simulink model "SF049A_LoaMgr"  (R2013b)
settings: Solver=FixedStepDiscrete  SolverMode=SingleTasking  StartTime=0.0  StopTime=1  FixedStep=0.002  RelTol=1e-3
values from neighbouring files (symbols this model uses):
  CURRMEASLOAMTGTNMASK_CNT_U08 = DataDict.Constant    [SF049A_LoaMgr_DataDict.m]
  IVTRLOAMTGTNMASK_CNT_U08 = DataDict.Constant    [SF049A_LoaMgr_DataDict.m]
  LOAMAXSLEW_ULSPERSEC_F32 = DataDict.Constant    [SF049A_LoaMgr_DataDict.m]
  LoaMgrCurrIvtrMtgtnRate = DataDict.Calibration    [SF049A_LoaMgr_DataDict.m]
  LoaMgrCurrIvtrMtgtnSca = DataDict.Calibration    [SF049A_LoaMgr_DataDict.m]
  LoaMgrCurrIvtrMtgtnScaZeroEna = DataDict.Calibration    [SF049A_LoaMgr_DataDict.m]
  LoaMgrCurrMeasIdptSig0Resp = DataDict.Calibration    [SF049A_LoaMgr_DataDict.m]
  LoaMgrCurrMeasIdptSig1Resp = DataDict.Calibration    [SF049A_LoaMgr_DataDict.m]
  LoaMgrCurrMeasIdptSig2Resp = DataDict.Calibration    [SF049A_LoaMgr_DataDict.m]
  LoaMgrCurrMeasIdptSigFltThd = DataDict.Calibration    [SF049A_LoaMgr_DataDict.m]
  LoaMgrCurrMeasMtgtnRate = DataDict.Calibration    [SF049A_LoaMgr_DataDict.m]
  LoaMgrCurrMeasMtgtnSca = DataDict.Calibration    [SF049A_LoaMgr_DataDict.m]
  LoaMgrCurrMeasMtgtnScaZeroEna = DataDict.Calibration    [SF049A_LoaMgr_DataDict.m]
  LoaMgrFadeOutStRate = DataDict.Calibration    [SF049A_LoaMgr_DataDict.m]
  LoaMgrHwTqIdptSig0NoTqLoaResp = DataDict.Calibration    [SF049A_LoaMgr_DataDict.m]
  LoaMgrHwTqIdptSig1NoTqLoaResp = DataDict.Calibration    [SF049A_LoaMgr_DataDict.m]
  LoaMgrHwTqIdptSig2Resp = DataDict.Calibration    [SF049A_LoaMgr_DataDict.m]
  LoaMgrHwTqIdptSig4Resp = DataDict.Calibration    [SF049A_LoaMgr_DataDict.m]
  LoaMgrHwTqIdptSigFltThd = DataDict.Calibration    [SF049A_LoaMgr_DataDict.m]
  LoaMgrHwTqLoaAvlResp = DataDict.Calibration    [SF049A_LoaMgr_DataDict.m]
  LoaMgrIvtrIdptSig0Resp = DataDict.Calibration    [SF049A_LoaMgr_DataDict.m]
  LoaMgrIvtrIdptSig1Resp = DataDict.Calibration    [SF049A_LoaMgr_DataDict.m]
  LoaMgrIvtrIdptSig2Resp = DataDict.Calibration    [SF049A_LoaMgr_DataDict.m]
  LoaMgrIvtrIdptSigFltThd = DataDict.Calibration    [SF049A_LoaMgr_DataDict.m]
  LoaMgrIvtrMtgtnRate = DataDict.Calibration    [SF049A_LoaMgr_DataDict.m]
  LoaMgrIvtrMtgtnSca = DataDict.Calibration    [SF049A_LoaMgr_DataDict.m]
  LoaMgrIvtrMtgtnScaZeroEna = DataDict.Calibration    [SF049A_LoaMgr_DataDict.m]
  LoaMgrLimdStRate = DataDict.Calibration    [SF049A_LoaMgr_DataDict.m]
  LoaMgrLimdStSca = DataDict.Calibration    [SF049A_LoaMgr_DataDict.m]
  LoaMgrMotAgAvlSnsrlsResp = DataDict.Calibration    [SF049A_LoaMgr_DataDict.m]
  LoaMgrMotAgIdptSig0NoSnsrlsResp = DataDict.Calibration    [SF049A_LoaMgr_DataDict.m]
  LoaMgrMotAgIdptSig1NoSnsrlsResp = DataDict.Calibration    [SF049A_LoaMgr_DataDict.m]
  LoaMgrMotAgIdptSig2Resp = DataDict.Calibration    [SF049A_LoaMgr_DataDict.m]
  LoaMgrMotAgIdptSig3Resp = DataDict.Calibration    [SF049A_LoaMgr_DataDict.m]
  LoaMgrMotAgIdptSigFltThd = DataDict.Calibration    [SF049A_LoaMgr_DataDict.m]
  LoaMgrMotAgMtgtnRate = DataDict.Calibration    [SF049A_LoaMgr_DataDict.m]
  LoaMgrMotAgMtgtnSca = DataDict.Calibration    [SF049A_LoaMgr_DataDict.m]
  LoaMgrMotAgMtgtnScaZeroEna = DataDict.Calibration    [SF049A_LoaMgr_DataDict.m]
  LOASCAONE_ULS_F32 = DataDict.Constant    [SF049A_LoaMgr_DataDict.m]
  LOASCAZERO_ULS_F32 = DataDict.Constant    [SF049A_LoaMgr_DataDict.m]
  LOASTIMDTSHTDWN_CNT_U08 = DataDict.Constant    [SF049A_LoaMgr_DataDict.m]
  LOASTNORM_CNT_U08 = DataDict.Constant    [SF049A_LoaMgr_DataDict.m]
  LOASTSWMTGTN_CNT_U08 = DataDict.Constant    [SF049A_LoaMgr_DataDict.m]
  MAXCURRMEASIDPTSIGALLWD_CNT_U08 = DataDict.Constant    [SF049A_LoaMgr_DataDict.m]
  MAXHWTQIDPTSIGALLWD_CNT_U08 = DataDict.Constant    [SF049A_LoaMgr_DataDict.m]
  MAXIVTRIDPTSIGALLWD_CNT_U08 = DataDict.Constant    [SF049A_LoaMgr_DataDict.m]
  MAXMOTAGMECLIDPTSIGALLWD_CNT_U08 = DataDict.Constant    [SF049A_LoaMgr_DataDict.m]
  NODEBSTEP_CNT_U16 = DataDict.Constant    [SF049A_LoaMgr_DataDict.m]
undefined symbols (not defined in the file or in its folder): LoaSt1, NtcNr1, NtcSts1, SigQlfr1
libraries: simulink x43, NxtrMin x4, NxtrMax x4, NxtrLim x2
(part 6 of 8)

== system SF049A_LoaMgr/LoaMgr/LoaMgrPer1/Assign_Scale/SwMtgtn/MaskBooleans ==
  note: Mask the booleans as integers with power of two values.  Add them to generate a temporary
      | variable whose value represents each unique combination of the two boolean inputs.
  note: value = 1
  note: value = 2
  CurrMeasLoaMtgtnEna : Inport  RequirementInfo="{'linktype_rmi_doors' '0000bab3 (/E-STEER Core/SubSystem Specifications/Application Functions/SF049A Loss of Assist Manager)' '#SF049A_103' 'true' 'REQ:  SF049A_103' '' } %GIDa_7d15856d_f4e8_4151_8a92_f8dddbad85bf"
  IvtrLoaMtgtnEna : Inport  RequirementInfo="{'linktype_rmi_doors' '0000bab3 (/E-STEER Core/SubSystem Specifications/Application Functions/SF049A Loss of Assist Manager)' '#SF049A_103' 'true' 'REQ:  SF049A_103' '' } %GIDa_3c6fad4d_d019_40b9_bac4_3461dd4c79ca"  Port=2
  Add1 : Sum  RequirementInfo="{'linktype_rmi_doors' '0000bab3 (/E-STEER Core/SubSystem Specifications/Application Functions/SF049A Loss of Assist Manager)' '#SF049A_103' 'true' 'REQ:  SF049A_103' '' } %GIDa_59e37b96_814a_4847_af89_aab73724b399"
  Constant1 : Constant  RequirementInfo="{'linktype_rmi_doors' '0000bab3 (/E-STEER Core/SubSystem Specifications/Application Functions/SF049A Loss of Assist Manager)' '#SF049A_103' 'true' 'REQ:  SF049A_103' '' } %GIDa_9cc5ef5a_9d6b_4095_b8f9_cefe803efae2"  Value=CURRMEASLOAMTGTNMASK_CNT_U08
  Constant2 : Constant  RequirementInfo="{'linktype_rmi_doors' '0000bab3 (/E-STEER Core/SubSystem Specifications/Application Functions/SF049A Loss of Assist Manager)' '#SF049A_103' 'true' 'REQ:  SF049A_103' '' } %GIDa_4ef13982_6e67_4a46_9ee5_090525304802"  Value=0  OutDataTypeStr=uint8
  Constant5 : Constant  RequirementInfo="{'linktype_rmi_doors' '0000bab3 (/E-STEER Core/SubSystem Specifications/Application Functions/SF049A Loss of Assist Manager)' '#SF049A_103' 'true' 'REQ:  SF049A_103' '' } %GIDa_6abb1c14_595b_4309_be03_a8ad2d5b3cff"  Value=IVTRLOAMTGTNMASK_CNT_U08
  Constant6 : Constant  RequirementInfo="{'linktype_rmi_doors' '0000bab3 (/E-STEER Core/SubSystem Specifications/Application Functions/SF049A Loss of Assist Manager)' '#SF049A_103' 'true' 'REQ:  SF049A_103' '' } %GIDa_a3f4c951_2fc7_4eeb_93ac_275886e553ed"  Value=0  OutDataTypeStr=uint8
  CopyRight2 : Subsystem  Description=|  mask(Copyright Information){none=on}
      | Copyright info block.                                               
      |                                                                     
      | Place copyright information at the top of every subsystem in design.
      mask prompts: none "No parameters"
      mask help: Place copyright information at the top of every subsystem in design.
      mask Display:
      | NxtrConf = 'Nexteer Confidential';
      | 
      | sys = bdroot; %handle for the current model ("system")
      | first = get_param(sys,'Created');
      | first = first(end-3:end);  %year is last four digits
      | 
      | last = get_param(sys,'LastModifiedDate');
      | if isempty(last)
      |     last = datestr(now,'yyyy');
      | else
      |     last = last(end-3:end);
      | end
      | 
      | if strcmp(first,last)
      |     fprintf('%s -- Copyright %s Nexteer',NxtrConf,first)
      | else
      |     fprintf('%s -- %s%s- %s Nexteer',NxtrConf,char(169),first,last)
      | end
  CurrMeas_ELSE : Subsystem  RequirementInfo="{'linktype_rmi_doors' '0000bab3 (/E-STEER Core/SubSystem Specifications/Application Functions/SF049A Loss of Assist Manager)' '#SF049A_103' 'true' 'REQ:  SF049A_103' '' } %GIDa_e3728322_30c8_4789_85b4_eb67e9133913"  TreatAsAtomicUnit=on
      settings: RTWSystemCode=Inline
  CurrMeas_IF : If  RequirementInfo="{'linktype_rmi_doors' '0000bab3 (/E-STEER Core/SubSystem Specifications/Application Functions/SF049A Loss of Assist Manager)' '#SF049A_103' 'true' 'REQ:  SF049A_103' '' } %GIDa_77bfcb72_6128_4665_b6ff_49767e291a56"  IfExpression=u1
  CurrMeas_THEN : Subsystem  RequirementInfo="{'linktype_rmi_doors' '0000bab3 (/E-STEER Core/SubSystem Specifications/Application Functions/SF049A Loss of Assist Manager)' '#SF049A_103' 'true' 'REQ:  SF049A_103' '' } %GIDa_25ce50a4_485b_4826_82da_6733fc7f1e6a"  TreatAsAtomicUnit=on
      settings: RTWSystemCode=Inline
  Ivtr_ELSE : Subsystem  RequirementInfo="{'linktype_rmi_doors' '0000bab3 (/E-STEER Core/SubSystem Specifications/Application Functions/SF049A Loss of Assist Manager)' '#SF049A_103' 'true' 'REQ:  SF049A_103' '' } %GIDa_1a0f5d27_3f76_4ea9_ba5c_c7a13dbff074"  TreatAsAtomicUnit=on
      settings: RTWSystemCode=Inline
  Ivtr_IF : If  RequirementInfo="{'linktype_rmi_doors' '0000bab3 (/E-STEER Core/SubSystem Specifications/Application Functions/SF049A Loss of Assist Manager)' '#SF049A_103' 'true' 'REQ:  SF049A_103' '' } %GIDa_2fc27373_46b4_4279_b0be_961336ffcd3b"  IfExpression=u1
  Ivtr_THEN : Subsystem  RequirementInfo="{'linktype_rmi_doors' '0000bab3 (/E-STEER Core/SubSystem Specifications/Application Functions/SF049A Loss of Assist Manager)' '#SF049A_103' 'true' 'REQ:  SF049A_103' '' } %GIDa_fe15d6b8_8d33_4ecc_a7e3_b9dec06d86e3"  TreatAsAtomicUnit=on
      settings: RTWSystemCode=Inline
  Merge2 : Merge  RequirementInfo="{'linktype_rmi_doors' '0000bab3 (/E-STEER Core/SubSystem Specifications/Application Functions/SF049A Loss of Assist Manager)' '#SF049A_103' 'true' 'REQ:  SF049A_103' '' } %GIDa_f5d5fbc7_2dce_43b4_86d2_413418f86e1d"
  Merge3 : Merge  RequirementInfo="{'linktype_rmi_doors' '0000bab3 (/E-STEER Core/SubSystem Specifications/Application Functions/SF049A Loss of Assist Manager)' '#SF049A_103' 'true' 'REQ:  SF049A_103' '' } %GIDa_c04e4a70_d624_48e9_88a9_359c0b7d590c"
  VltgModSrc : Outport  RequirementInfo="{'linktype_rmi_doors' '0000bab3 (/E-STEER Core/SubSystem Specifications/Application Functions/SF049A Loss of Assist Manager)' '#SF049A_103' 'true' 'REQ:  SF049A_103' '' } %GIDa_aea9468e_dd14_43a7_b2a0_1c9441e50dad"
  wires:
  CurrMeas_IF/1 -> CurrMeas_THEN/Action
  CurrMeas_ELSE/1(Out1) -> Merge2/2
  Merge3/1 -> Add1/2
  Constant1/1 -> CurrMeas_THEN/1(In1)
  CurrMeas_THEN/1(Out1) -> Merge2/1
  Ivtr_THEN/1(Out1) -> Merge3/1
  Ivtr_ELSE/1(Out1) -> Merge3/2
  Constant6/1 -> Ivtr_ELSE/1(In1)
  Constant5/1 -> Ivtr_THEN/1(In1)
  Ivtr_IF/2 -> Ivtr_ELSE/Action
  Ivtr_IF/1 -> Ivtr_THEN/Action
  Constant2/1 -> CurrMeas_ELSE/1(In1)
  CurrMeas_IF/2 -> CurrMeas_ELSE/Action
  Merge2/1 -> Add1/1
  Add1/1 -> VltgModSrc/1
  CurrMeasLoaMtgtnEna/1 -> CurrMeas_IF/1
  IvtrLoaMtgtnEna/1 -> Ivtr_IF/1

== system SF049A_LoaMgr/LoaMgr/LoaMgrPer1/Assign_Scale/SwMtgtn/MotAgTrue ==
  note: IF cal is true and previous value is false THEN
      |      Target scale factor is Zero
      |      Slew rate is instantaneous
      | ELSE
      |      Target scale factor is a cal value
      |      Slew rate is a cal value
      | ENDIF
  note: We could only reach this routine when the new value is true
      | So if old value is false, it is our first time entering this block.
      | If the user wants to momentarily drop scale factor instantly to
      | zero, this transition from false to true is the time to do it.
  note: If we enter this block on the next loop, the state variable ("previous value") will already be
      | TRUE because of the current loop.  The user's calibrated scale factor and slew rate will
      | be used.  This means that the slew rate is applied whether the system is slewing down from
      | ONE or up from ZERO.
  PrevMotAgLoaMtgtnEn : Inport  RequirementInfo="{'linktype_rmi_doors' '0000bab3 (/E-STEER Core/SubSystem Specifications/Application Functions/SF049A Loss of Assist Manager)' '#SF049A_100' 'true' 'REQ:  SF049A_100' '' ; 'linktype_rmi_doors' '0000bab3 (/E-STEER Core/SubSystem Specifications/Application Functions/SF049A Loss of Assist Manager)' '#SF049A_101' 'true' 'REQ:  SF049A_101' '' } %GIDa_0fd04b14_63ff_4197_910e_67cb3aef4881"
  Action Port : ActionPort  ActionType=elseif
  Constant1 : Constant  RequirementInfo="{'linktype_rmi_doors' '0000bab3 (/E-STEER Core/SubSystem Specifications/Application Functions/SF049A Loss of Assist Manager)' '#SF049A_100' 'true' 'REQ:  SF049A_100' '' ; 'linktype_rmi_doors' '0000bab3 (/E-STEER Core/SubSystem Specifications/Application Functions/SF049A Loss of Assist Manager)' '#SF049A_101' 'true' 'REQ:  SF049A_101' '' ; 'linktype_rmi_doors' '0000bab3 (/E-STEER Core/SubSystem Specifications/Application Functions/SF049A Loss of Assist Manager)' '#SF049A_102' 'true' 'REQ:  SF049A_102' '' } %GIDa_1629df0d_a5ed_436d_b129_3d6428cde474"  Value=LoaMgrMotAgMtgtnRate
  Constant2 : Constant  RequirementInfo="{'linktype_rmi_doors' '0000bab3 (/E-STEER Core/SubSystem Specifications/Application Functions/SF049A Loss of Assist Manager)' '#SF049A_100' 'true' 'REQ:  SF049A_100' '' ; 'linktype_rmi_doors' '0000bab3 (/E-STEER Core/SubSystem Specifications/Application Functions/SF049A Loss of Assist Manager)' '#SF049A_101' 'true' 'REQ:  SF049A_101' '' } %GIDa_169a1e65_6b16_43ec_8e11_d2bb73154605"  Value=LOASCAZERO_ULS_F32
  Constant3 : Constant  RequirementInfo="{'linktype_rmi_doors' '0000bab3 (/E-STEER Core/SubSystem Specifications/Application Functions/SF049A Loss of Assist Manager)' '#SF049A_100' 'true' 'REQ:  SF049A_100' '' ; 'linktype_rmi_doors' '0000bab3 (/E-STEER Core/SubSystem Specifications/Application Functions/SF049A Loss of Assist Manager)' '#SF049A_101' 'true' 'REQ:  SF049A_101' '' } %GIDa_d994c6a4_4ee5_4a9c_b55f_408513d3dcf2"  Value=LOAMAXSLEW_ULSPERSEC_F32
  Constant4 : Constant  RequirementInfo="{'linktype_rmi_doors' '0000bab3 (/E-STEER Core/SubSystem Specifications/Application Functions/SF049A Loss of Assist Manager)' '#SF049A_100' 'true' 'REQ:  SF049A_100' '' ; 'linktype_rmi_doors' '0000bab3 (/E-STEER Core/SubSystem Specifications/Application Functions/SF049A Loss of Assist Manager)' '#SF049A_101' 'true' 'REQ:  SF049A_101' '' ; 'linktype_rmi_doors' '0000bab3 (/E-STEER Core/SubSystem Specifications/Application Functions/SF049A Loss of Assist Manager)' '#SF049A_102' 'true' 'REQ:  SF049A_102' '' } %GIDa_603b306d_a7bb_4140_a3cf_d5dad673a642"  Value=LoaMgrMotAgMtgtnScaZeroEna
  Constant6 : Constant  RequirementInfo="{'linktype_rmi_doors' '0000bab3 (/E-STEER Core/SubSystem Specifications/Application Functions/SF049A Loss of Assist Manager)' '#SF049A_100' 'true' 'REQ:  SF049A_100' '' ; 'linktype_rmi_doors' '0000bab3 (/E-STEER Core/SubSystem Specifications/Application Functions/SF049A Loss of Assist Manager)' '#SF049A_101' 'true' 'REQ:  SF049A_101' '' ; 'linktype_rmi_doors' '0000bab3 (/E-STEER Core/SubSystem Specifications/Application Functions/SF049A Loss of Assist Manager)' '#SF049A_102' 'true' 'REQ:  SF049A_102' '' } %GIDa_82c37d5e_f81f_456a_a4f0_c68450b59f50"  Value=LoaMgrMotAgMtgtnSca
  CopyRight2 : Subsystem  Description=|  mask(Copyright Information){none=on}
      | Copyright info block.                                               
      |                                                                     
      | Place copyright information at the top of every subsystem in design.
      mask prompts: none "No parameters"
      mask help: Place copyright information at the top of every subsystem in design.
      mask Display:
      | NxtrConf = 'Nexteer Confidential';
      | 
      | sys = bdroot; %handle for the current model ("system")
      | first = get_param(sys,'Created');
      | first = first(end-3:end);  %year is last four digits
      | 
      | last = get_param(sys,'LastModifiedDate');
      | if isempty(last)
      |     last = datestr(now,'yyyy');
      | else
      |     last = last(end-3:end);
      | end
      | 
      | if strcmp(first,last)
      |     fprintf('%s -- Copyright %s Nexteer',NxtrConf,first)
      | else
      |     fprintf('%s -- %s%s- %s Nexteer',NxtrConf,char(169),first,last)
      | end
  If : If  RequirementInfo="{'linktype_rmi_doors' '0000bab3 (/E-STEER Core/SubSystem Specifications/Application Functions/SF049A Loss of Assist Manager)' '#SF049A_100' 'true' 'REQ:  SF049A_100' '' ; 'linktype_rmi_doors' '0000bab3 (/E-STEER Core/SubSystem Specifications/Application Functions/SF049A Loss of Assist Manager)' '#SF049A_101' 'true' 'REQ:  SF049A_101' '' ; 'linktype_rmi_doors' '0000bab3 (/E-STEER Core/SubSystem Specifications/Application Functions/SF049A Loss of Assist Manager)' '#SF049A_102' 'true' 'REQ:  SF049A_102' '' } %GIDa_fc29df37_73fc_4c8b_907b_1c2b22027db1"  NumInputs=2  IfExpression=u2 & ~u1
  PassThru1 : Subsystem  RequirementInfo="{'linktype_rmi_doors' '0000bab3 (/E-STEER Core/SubSystem Specifications/Application Functions/SF049A Loss of Assist Manager)' '#SF049A_100' 'true' 'REQ:  SF049A_100' '' ; 'linktype_rmi_doors' '0000bab3 (/E-STEER Core/SubSystem Specifications/Application Functions/SF049A Loss of Assist Manager)' '#SF049A_101' 'true' 'REQ:  SF049A_101' '' } %GIDa_cb7f4f46_8edd_4e61_bb1b_7e1716ea7617"  TreatAsAtomicUnit=on
      settings: RTWSystemCode=Inline
  PassThru2 : Subsystem  RequirementInfo="{'linktype_rmi_doors' '0000bab3 (/E-STEER Core/SubSystem Specifications/Application Functions/SF049A Loss of Assist Manager)' '#SF049A_100' 'true' 'REQ:  SF049A_100' '' ; 'linktype_rmi_doors' '0000bab3 (/E-STEER Core/SubSystem Specifications/Application Functions/SF049A Loss of Assist Manager)' '#SF049A_101' 'true' 'REQ:  SF049A_101' '' ; 'linktype_rmi_doors' '0000bab3 (/E-STEER Core/SubSystem Specifications/Application Functions/SF049A Loss of Assist Manager)' '#SF049A_102' 'true' 'REQ:  SF049A_102' '' } %GIDa_90d2d5f0_7ad8_4bf2_8601_9d1a70b6f298"  TreatAsAtomicUnit=on
      settings: RTWSystemCode=Inline
  RateMerge : Merge  RequirementInfo="{'linktype_rmi_doors' '0000bab3 (/E-STEER Core/SubSystem Specifications/Application Functions/SF049A Loss of Assist Manager)' '#SF049A_100' 'true' 'REQ:  SF049A_100' '' ; 'linktype_rmi_doors' '0000bab3 (/E-STEER Core/SubSystem Specifications/Application Functions/SF049A Loss of Assist Manager)' '#SF049A_101' 'true' 'REQ:  SF049A_101' '' ; 'linktype_rmi_doors' '0000bab3 (/E-STEER Core/SubSystem Specifications/Application Functions/SF049A Loss of Assist Manager)' '#SF049A_102' 'true' 'REQ:  SF049A_102' '' } %GIDa_6714992d_c037_47fa_9050_dcbd7c2a04f8"
  ScaMerge : Merge  RequirementInfo="{'linktype_rmi_doors' '0000bab3 (/E-STEER Core/SubSystem Specifications/Application Functions/SF049A Loss of Assist Manager)' '#SF049A_100' 'true' 'REQ:  SF049A_100' '' ; 'linktype_rmi_doors' '0000bab3 (/E-STEER Core/SubSystem Specifications/Application Functions/SF049A Loss of Assist Manager)' '#SF049A_101' 'true' 'REQ:  SF049A_101' '' ; 'linktype_rmi_doors' '0000bab3 (/E-STEER Core/SubSystem Specifications/Application Functions/SF049A Loss of Assist Manager)' '#SF049A_102' 'true' 'REQ:  SF049A_102' '' } %GIDa_2de96d30_e63b_4315_8361_f9ffb9bd39cf"
  Sca : Outport  RequirementInfo="{'linktype_rmi_doors' '0000bab3 (/E-STEER Core/SubSystem Specifications/Application Functions/SF049A Loss of Assist Manager)' '#SF049A_100' 'true' 'REQ:  SF049A_100' '' ; 'linktype_rmi_doors' '0000bab3 (/E-STEER Core/SubSystem Specifications/Application Functions/SF049A Loss of Assist Manager)' '#SF049A_101' 'true' 'REQ:  SF049A_101' '' ; 'linktype_rmi_doors' '0000bab3 (/E-STEER Core/SubSystem Specifications/Application Functions/SF049A Loss of Assist Manager)' '#SF049A_102' 'true' 'REQ:  SF049A_102' '' } %GIDa_66450784_8427_49b3_b12c_c08c02cce883"
  Rate : Outport  RequirementInfo="{'linktype_rmi_doors' '0000bab3 (/E-STEER Core/SubSystem Specifications/Application Functions/SF049A Loss of Assist Manager)' '#SF049A_100' 'true' 'REQ:  SF049A_100' '' ; 'linktype_rmi_doors' '0000bab3 (/E-STEER Core/SubSystem Specifications/Application Functions/SF049A Loss of Assist Manager)' '#SF049A_101' 'true' 'REQ:  SF049A_101' '' ; 'linktype_rmi_doors' '0000bab3 (/E-STEER Core/SubSystem Specifications/Application Functions/SF049A Loss of Assist Manager)' '#SF049A_102' 'true' 'REQ:  SF049A_102' '' } %GIDa_de956b84_d897_4d44_8482_e2d99c11e837"  Port=2
  wires:
  ScaMerge/1 -> Sca/1
  RateMerge/1 -> Rate/1
  PrevMotAgLoaMtgtnEn/1 -> If/1
  Constant4/1 -> If/2
  Constant2/1 -> PassThru1/1(In1)
  Constant3/1 -> PassThru1/2(In2)
  Constant6/1 -> PassThru2/1(In1)
  Constant1/1 -> PassThru2/2(In2)
  If/1 -> PassThru1/Action
  If/2 -> PassThru2/Action
  PassThru1/1(Sca) -> ScaMerge/1
  PassThru1/2(Rate) -> RateMerge/1
  PassThru2/1(Sca) -> ScaMerge/2
  PassThru2/2(Rate) -> RateMerge/2

== system SF049A_LoaMgr/LoaMgr/LoaMgrPer1/Assign_Scale/SwMtgtn/OthersTrue ==
  note: Value Assignments
      |   0  neither enabled (shouldn't get here if this is true)
      |   1  MotCurrLoaMtgtnEn
      |   2  IvtrLoaMtgtnEn
      |   3  both enabled
  VltgModSrc : Inport  RequirementInfo="{'linktype_rmi_doors' '0000bab3 (/E-STEER Core/SubSystem Specifications/Application Functions/SF049A Loss of Assist Manager)' '#SF049A_107' 'true' 'REQ:  SF049A_107' '' ; 'linktype_rmi_doors' '0000bab3 (/E-STEER Core/SubSystem Specifications/Application Functions/SF049A Loss of Assist Manager)' '#SF049A_108' 'true' 'REQ:  SF049A_108' '' } %GIDa_243c8b93_8009_4634_83ee_a48e40a4d53d"
  PrevVltgModSrc : Inport  RequirementInfo="{'linktype_rmi_doors' '0000bab3 (/E-STEER Core/SubSystem Specifications/Application Functions/SF049A Loss of Assist Manager)' '#SF049A_107' 'true' 'REQ:  SF049A_107' '' } %GIDa_40fea561_cefb_4f51_897f_c9ee51d9a5ab"  Port=2
  Action Port : ActionPort  ActionType=else
  CopyRight2 : Subsystem  Description=|  mask(Copyright Information){none=on}
      | Copyright info block.                                               
      |                                                                     
      | Place copyright information at the top of every subsystem in design.
      mask prompts: none "No parameters"
      mask help: Place copyright information at the top of every subsystem in design.
      mask Display:
      | NxtrConf = 'Nexteer Confidential';
      | 
      | sys = bdroot; %handle for the current model ("system")
      | first = get_param(sys,'Created');
      | first = first(end-3:end);  %year is last four digits
      | 
      | last = get_param(sys,'LastModifiedDate');
      | if isempty(last)
      |     last = datestr(now,'yyyy');
      | else
      |     last = last(end-3:end);
      | end
      | 
      | if strcmp(first,last)
      |     fprintf('%s -- Copyright %s Nexteer',NxtrConf,first)
      | else
      |     fprintf('%s -- %s%s- %s Nexteer',NxtrConf,char(169),first,last)
      | end
  CurrIvtr : Subsystem  TreatAsAtomicUnit=on
  CurrOnly : Subsystem  TreatAsAtomicUnit=on
  DidItChange : RelationalOperator  RequirementInfo="{'linktype_rmi_doors' '0000bab3 (/E-STEER Core/SubSystem Specifications/Application Functions/SF049A Loss of Assist Manager)' '#SF049A_107' 'true' 'REQ:  SF049A_107' '' } %GIDa_a97e9b3f_1cf1_48d9_a13d_5fa845d4858e"  Operator=~=  OutDataTypeStr=boolean
  Invalid_Number : Subsystem  TreatAsAtomicUnit=on
  IvtrOnly : Subsystem  TreatAsAtomicUnit=on
  RateMerge : Merge  RequirementInfo="{'linktype_rmi_doors' '0000bab3 (/E-STEER Core/SubSystem Specifications/Application Functions/SF049A Loss of Assist Manager)' '#SF049A_107' 'true' 'REQ:  SF049A_107' '' ; 'linktype_rmi_doors' '0000bab3 (/E-STEER Core/SubSystem Specifications/Application Functions/SF049A Loss of Assist Manager)' '#SF049A_108' 'true' 'REQ:  SF049A_108' '' } %GIDa_d7078a40_1d9f_473b_ab87_88c57d786196"  Inputs=4
  ScaMerge : Merge  RequirementInfo="{'linktype_rmi_doors' '0000bab3 (/E-STEER Core/SubSystem Specifications/Application Functions/SF049A Loss of Assist Manager)' '#SF049A_107' 'true' 'REQ:  SF049A_107' '' ; 'linktype_rmi_doors' '0000bab3 (/E-STEER Core/SubSystem Specifications/Application Functions/SF049A Loss of Assist Manager)' '#SF049A_108' 'true' 'REQ:  SF049A_108' '' } %GIDa_6e3a33d1_a1d1_453c_8d35_8e2fe46f9b59"  Inputs=4
  Switch Case : SwitchCase  RequirementInfo="{'linktype_rmi_doors' '0000bab3 (/E-STEER Core/SubSystem Specifications/Application Functions/SF049A Loss of Assist Manager)' '#SF049A_107' 'true' 'REQ:  SF049A_107' '' ; 'linktype_rmi_doors' '0000bab3 (/E-STEER Core/SubSystem Specifications/Application Functions/SF049A Loss of Assist Manager)' '#SF049A_108' 'true' 'REQ:  SF049A_108' '' } %GIDa_18df147d_a7b4_42b2_8f1b_b1aa839e2938"  CaseConditions={1,2,3}
  Sca : Outport  RequirementInfo="{'linktype_rmi_doors' '0000bab3 (/E-STEER Core/SubSystem Specifications/Application Functions/SF049A Loss of Assist Manager)' '#SF049A_107' 'true' 'REQ:  SF049A_107' '' ; 'linktype_rmi_doors' '0000bab3 (/E-STEER Core/SubSystem Specifications/Application Functions/SF049A Loss of Assist Manager)' '#SF049A_108' 'true' 'REQ:  SF049A_108' '' } %GIDa_68215d0b_0b2e_42f4_9200_8bd549c9ecdb"
  Rate : Outport  RequirementInfo="{'linktype_rmi_doors' '0000bab3 (/E-STEER Core/SubSystem Specifications/Application Functions/SF049A Loss of Assist Manager)' '#SF049A_107' 'true' 'REQ:  SF049A_107' '' ; 'linktype_rmi_doors' '0000bab3 (/E-STEER Core/SubSystem Specifications/Application Functions/SF049A Loss of Assist Manager)' '#SF049A_108' 'true' 'REQ:  SF049A_108' '' } %GIDa_ca053ee3_7b58_44c6_b1ad_17b82af4b7a9"  Port=2
  wires:
  VltgModSrc/1 -> DidItChange/1, Switch Case/1
  ScaMerge/1 -> Sca/1
  RateMerge/1 -> Rate/1
  PrevVltgModSrc/1 -> DidItChange/2
  DidItChange/1 -> [Changed]
  [Changed] -> CurrOnly/1(NewValFlg)
  [Changed] -> IvtrOnly/1(NewValFlg)
  [Changed] -> CurrIvtr/1(NewValFlg)
  Switch Case/1 -> CurrOnly/Action
  Switch Case/2 -> IvtrOnly/Action
  Switch Case/3 -> CurrIvtr/Action
  Switch Case/4 -> Invalid_Number/Action
  CurrOnly/1(Sca) -> ScaMerge/1
  IvtrOnly/1(Sca) -> ScaMerge/2
  CurrIvtr/1(Sca) -> ScaMerge/3
  Invalid_Number/1(Sca) -> ScaMerge/4
  CurrOnly/2(Rate) -> RateMerge/1
  IvtrOnly/2(Rate) -> RateMerge/2
  CurrIvtr/2(Rate) -> RateMerge/3
  Invalid_Number/2(Rate) -> RateMerge/4

== system SF049A_LoaMgr/LoaMgr/LoaMgrPer1/Latch_Inputs/RngLimCurrMeasIdptSig/Allw ==
  In1 : Inport
  Action Port : ActionPort  ActionType=else
  Out1 : Outport
  wires:
  In1/1 -> Out1/1

== system SF049A_LoaMgr/LoaMgr/LoaMgrPer1/Latch_Inputs/RngLimCurrMeasIdptSig/CopyRight2 ==

== system SF049A_LoaMgr/LoaMgr/LoaMgrPer1/Latch_Inputs/RngLimCurrMeasIdptSig/DftVal ==
  In1 : Inport
  Action Port : ActionPort  ActionType=then
  Out2 : Outport
  wires:
  In1/1 -> Out2/1

== system SF049A_LoaMgr/LoaMgr/LoaMgrPer1/Latch_Inputs/RngLimHwTqIdptSig/Allw ==
  In1 : Inport
  Action Port : ActionPort  ActionType=else
  Out1 : Outport
  wires:
  In1/1 -> Out1/1

== system SF049A_LoaMgr/LoaMgr/LoaMgrPer1/Latch_Inputs/RngLimHwTqIdptSig/CopyRight2 ==

== system SF049A_LoaMgr/LoaMgr/LoaMgrPer1/Latch_Inputs/RngLimHwTqIdptSig/DftVal ==
  In1 : Inport
  Action Port : ActionPort  ActionType=then
  Out2 : Outport
  wires:
  In1/1 -> Out2/1

== system SF049A_LoaMgr/LoaMgr/LoaMgrPer1/Latch_Inputs/RngLimMotAgMecIdptSig/Allw ==
  In1 : Inport
  Action Port : ActionPort  ActionType=else
  Out1 : Outport
  wires:
  In1/1 -> Out1/1

== system SF049A_LoaMgr/LoaMgr/LoaMgrPer1/Latch_Inputs/RngLimMotAgMecIdptSig/CopyRight2 ==

== system SF049A_LoaMgr/LoaMgr/LoaMgrPer1/Latch_Inputs/RngLimMotAgMecIdptSig/DftVal ==
  In1 : Inport
  Action Port : ActionPort  ActionType=then
  Out2 : Outport
  wires:
  In1/1 -> Out2/1

== system SF049A_LoaMgr/LoaMgr/LoaMgrPer1/Request_Responses/CurrMeasResp/CopyRight2 ==

== system SF049A_LoaMgr/LoaMgr/LoaMgrPer1/Request_Responses/CurrMeasResp/Two ==
  Sig2Resp : Inport
  Two : ActionPort  ActionType=case
  CopyRight2 : Subsystem  Description=|  mask(Copyright Information){none=on}
      | Copyright info block.                                               
      |                                                                     
      | Place copyright information at the top of every subsystem in design.
      mask prompts: none "No parameters"
      mask help: Place copyright information at the top of every subsystem in design.
      mask Display:
      | NxtrConf = 'Nexteer Confidential';
      | 
      | sys = bdroot; %handle for the current model ("system")
      | first = get_param(sys,'Created');
      | first = first(end-3:end);  %year is last four digits
      | 
      | last = get_param(sys,'LastModifiedDate');
      | if isempty(last)
      |     last = datestr(now,'yyyy');
      | else
      |     last = last(end-3:end);
      | end
      | 
      | if strcmp(first,last)
      |     fprintf('%s -- Copyright %s Nexteer',NxtrConf,first)
      | else
      |     fprintf('%s -- %s%s- %s Nexteer',NxtrConf,char(169),first,last)
      | end
  CurrMeasResp : Outport
  wires:
  Sig2Resp/1 -> CurrMeasResp/1

== system SF049A_LoaMgr/LoaMgr/LoaMgrPer1/Request_Responses/CurrMeasResp/Zero_or_Invalid ==
  Sig0Resp : Inport
  Default : ActionPort  ActionType=default
  CopyRight2 : Subsystem  Description=|  mask(Copyright Information){none=on}
      | Copyright info block.                                               
      |                                                                     
      | Place copyright information at the top of every subsystem in design.
      mask prompts: none "No parameters"
      mask help: Place copyright information at the top of every subsystem in design.
      mask Display:
      | NxtrConf = 'Nexteer Confidential';
      | 
      | sys = bdroot; %handle for the current model ("system")
      | first = get_param(sys,'Created');
      | first = first(end-3:end);  %year is last four digits
      | 
      | last = get_param(sys,'LastModifiedDate');
      | if isempty(last)
      |     last = datestr(now,'yyyy');
      | else
      |     last = last(end-3:end);
      | end
      | 
      | if strcmp(first,last)
      |     fprintf('%s -- Copyright %s Nexteer',NxtrConf,first)
      | else
      |     fprintf('%s -- %s%s- %s Nexteer',NxtrConf,char(169),first,last)
      | end
  CurrMeasResp : Outport
  wires:
  Sig0Resp/1 -> CurrMeasResp/1

== system SF049A_LoaMgr/LoaMgr/LoaMgrPer1/Request_Responses/CurrMeasResp/one ==
  Sig1Resp : Inport
  one : ActionPort  ActionType=case
  CopyRight2 : Subsystem  Description=|  mask(Copyright Information){none=on}
      | Copyright info block.                                               
      |                                                                     
      | Place copyright information at the top of every subsystem in design.
      mask prompts: none "No parameters"
      mask help: Place copyright information at the top of every subsystem in design.
      mask Display:
      | NxtrConf = 'Nexteer Confidential';
      | 
      | sys = bdroot; %handle for the current model ("system")
      | first = get_param(sys,'Created');
      | first = first(end-3:end);  %year is last four digits
      | 
      | last = get_param(sys,'LastModifiedDate');
      | if isempty(last)
      |     last = datestr(now,'yyyy');
      | else
      |     last = last(end-3:end);
      | end
      | 
      | if strcmp(first,last)
      |     fprintf('%s -- Copyright %s Nexteer',NxtrConf,first)
      | else
      |     fprintf('%s -- %s%s- %s Nexteer',NxtrConf,char(169),first,last)
      | end
  CurrMeasResp : Outport
  wires:
  Sig1Resp/1 -> CurrMeasResp/1

== system SF049A_LoaMgr/LoaMgr/LoaMgrPer1/Request_Responses/HwTqResp/CopyRight2 ==

== system SF049A_LoaMgr/LoaMgr/LoaMgrPer1/Request_Responses/HwTqResp/Four ==
  cal : Inport
  Four : ActionPort  ActionType=case
  CopyRight2 : Subsystem  Description=|  mask(Copyright Information){none=on}
      | Copyright info block.                                               
      |                                                                     
      | Place copyright information at the top of every subsystem in design.
      mask prompts: none "No parameters"
      mask help: Place copyright information at the top of every subsystem in design.
      mask Display:
      | NxtrConf = 'Nexteer Confidential';
      | 
      | sys = bdroot; %handle for the current model ("system")
      | first = get_param(sys,'Created');
      | first = first(end-3:end);  %year is last four digits
      | 
      | last = get_param(sys,'LastModifiedDate');
      | if isempty(last)
      |     last = datestr(now,'yyyy');
      | else
      |     last = last(end-3:end);
      | end
      | 
      | if strcmp(first,last)
      |     fprintf('%s -- Copyright %s Nexteer',NxtrConf,first)
      | else
      |     fprintf('%s -- %s%s- %s Nexteer',NxtrConf,char(169),first,last)
      | end
  HwTqResp : Outport
  wires:
  cal/1 -> HwTqResp/1

== system SF049A_LoaMgr/LoaMgr/LoaMgrPer1/Request_Responses/HwTqResp/Two ==
  cal : Inport
  Two : ActionPort  ActionType=case
  CopyRight2 : Subsystem  Description=|  mask(Copyright Information){none=on}
      | Copyright info block.                                               
      |                                                                     
      | Place copyright information at the top of every subsystem in design.
      mask prompts: none "No parameters"
      mask help: Place copyright information at the top of every subsystem in design.
      mask Display:
      | NxtrConf = 'Nexteer Confidential';
      | 
      | sys = bdroot; %handle for the current model ("system")
      | first = get_param(sys,'Created');
      | first = first(end-3:end);  %year is last four digits
      | 
      | last = get_param(sys,'LastModifiedDate');
      | if isempty(last)
      |     last = datestr(now,'yyyy');
      | else
      |     last = last(end-3:end);
      | end
      | 
      | if strcmp(first,last)
      |     fprintf('%s -- Copyright %s Nexteer',NxtrConf,first)
      | else
      |     fprintf('%s -- %s%s- %s Nexteer',NxtrConf,char(169),first,last)
      | end
  HwTqResp : Outport
  wires:
  cal/1 -> HwTqResp/1

== system SF049A_LoaMgr/LoaMgr/LoaMgrPer1/Request_Responses/HwTqResp/Zero_or_Invalid ==
  TqLoaAvlResp : Inport
  Sig0NoTqLoaResp : Inport  Port=2
  TqLoaAvl : Inport  Port=3
  default : ActionPort  ActionType=default
  " " : Merge  RequirementInfo="{'linktype_rmi_doors' '0000bab3 (/E-STEER Core/SubSystem Specifications/Application Functions/SF049A Loss of Assist Manager)' '#SF049A_183' 'true' 'REQ:  SF049A_183' '' } %GIDa_a37e97d9_ee30_4c60_a863_730feb7f147f"
  CopyRight2 : Subsystem  Description=|  mask(Copyright Information){none=on}
      | Copyright info block.                                               
      |                                                                     
      | Place copyright information at the top of every subsystem in design.
      mask prompts: none "No parameters"
      mask help: Place copyright information at the top of every subsystem in design.
      mask Display:
      | NxtrConf = 'Nexteer Confidential';
      | 
      | sys = bdroot; %handle for the current model ("system")
      | first = get_param(sys,'Created');
      | first = first(end-3:end);  %year is last four digits
      | 
      | last = get_param(sys,'LastModifiedDate');
      | if isempty(last)
      |     last = datestr(now,'yyyy');
      | else
      |     last = last(end-3:end);
      | end
      | 
      | if strcmp(first,last)
      |     fprintf('%s -- Copyright %s Nexteer',NxtrConf,first)
      | else
      |     fprintf('%s -- %s%s- %s Nexteer',NxtrConf,char(169),first,last)
      | end
  Ivtr1Inactv_IF : If  RequirementInfo="{'linktype_rmi_doors' '0000bab3 (/E-STEER Core/SubSystem Specifications/Application Functions/SF049A Loss of Assist Manager)' '#SF049A_183' 'true' 'REQ:  SF049A_183' '' } %GIDa_2c9a8f4a_0f81_433e_a9ea_f88b2c0f52c9"  IfExpression=u1
  cal1 : Subsystem  RequirementInfo="{'linktype_rmi_doors' '0000bab3 (/E-STEER Core/SubSystem Specifications/Application Functions/SF049A Loss of Assist Manager)' '#SF049A_183' 'true' 'REQ:  SF049A_183' '' } %GIDa_79157d3e_063b_499f_a64c_457717d16ee5"  TreatAsAtomicUnit=on
      settings: RTWSystemCode=Inline
  cal2 : Subsystem  RequirementInfo="{'linktype_rmi_doors' '0000bab3 (/E-STEER Core/SubSystem Specifications/Application Functions/SF049A Loss of Assist Manager)' '#SF049A_183' 'true' 'REQ:  SF049A_183' '' } %GIDa_ecacb95a_1b4b_4f00_8700_d26d9f74486f"  TreatAsAtomicUnit=on
      settings: RTWSystemCode=Inline
  HwTqResp : Outport
  wires:
  Ivtr1Inactv_IF/2 -> cal2/Action
  Ivtr1Inactv_IF/1 -> cal1/Action
  cal2/1(Out1) -> " "/2
  TqLoaAvl/1 -> Ivtr1Inactv_IF/1
  cal1/1(Out2) -> " "/1
  TqLoaAvlResp/1 -> cal1/1(In1)
  Sig0NoTqLoaResp/1 -> cal2/1(In1)
  " "/1 -> HwTqResp/1

== system SF049A_LoaMgr/LoaMgr/LoaMgrPer1/Request_Responses/HwTqResp/one ==
  TqLoaAvlResp : Inport
  Sig1NoTqLoaResp : Inport  Port=2
  TqLoaAvl : Inport  Port=3
  one : ActionPort  ActionType=case
  " " : Merge  RequirementInfo="{'linktype_rmi_doors' '0000bab3 (/E-STEER Core/SubSystem Specifications/Application Functions/SF049A Loss of Assist Manager)' '#SF049A_183' 'true' 'REQ:  SF049A_183' '' } %GIDa_020f06ab_c766_4250_a2ae_03688a84ecec"
  CopyRight2 : Subsystem  Description=|  mask(Copyright Information){none=on}
      | Copyright info block.                                               
      |                                                                     
      | Place copyright information at the top of every subsystem in design.
      mask prompts: none "No parameters"
      mask help: Place copyright information at the top of every subsystem in design.
      mask Display:
      | NxtrConf = 'Nexteer Confidential';
      | 
      | sys = bdroot; %handle for the current model ("system")
      | first = get_param(sys,'Created');
      | first = first(end-3:end);  %year is last four digits
      | 
      | last = get_param(sys,'LastModifiedDate');
      | if isempty(last)
      |     last = datestr(now,'yyyy');
      | else
      |     last = last(end-3:end);
      | end
      | 
      | if strcmp(first,last)
      |     fprintf('%s -- Copyright %s Nexteer',NxtrConf,first)
      | else
      |     fprintf('%s -- %s%s- %s Nexteer',NxtrConf,char(169),first,last)
      | end
  Ivtr1Inactv_IF : If  RequirementInfo="{'linktype_rmi_doors' '0000bab3 (/E-STEER Core/SubSystem Specifications/Application Functions/SF049A Loss of Assist Manager)' '#SF049A_183' 'true' 'REQ:  SF049A_183' '' } %GIDa_bfa4b9ae_a722_4e43_97e6_68483ea7e917"  IfExpression=u1
  cal1 : Subsystem  RequirementInfo="{'linktype_rmi_doors' '0000bab3 (/E-STEER Core/SubSystem Specifications/Application Functions/SF049A Loss of Assist Manager)' '#SF049A_183' 'true' 'REQ:  SF049A_183' '' } %GIDa_692e5b5e_1cf9_4f54_8533_843c41e62cbe"  TreatAsAtomicUnit=on
      settings: RTWSystemCode=Inline
  cal2 : Subsystem  RequirementInfo="{'linktype_rmi_doors' '0000bab3 (/E-STEER Core/SubSystem Specifications/Application Functions/SF049A Loss of Assist Manager)' '#SF049A_183' 'true' 'REQ:  SF049A_183' '' } %GIDa_fd1696d7_8733_4f3c_a75e_abe6679e3523"  TreatAsAtomicUnit=on
      settings: RTWSystemCode=Inline
  HwTqResp : Outport
  wires:
  Ivtr1Inactv_IF/2 -> cal2/Action
  Ivtr1Inactv_IF/1 -> cal1/Action
  cal2/1(Out1) -> " "/2
  TqLoaAvl/1 -> Ivtr1Inactv_IF/1
  cal1/1(Out2) -> " "/1
  TqLoaAvlResp/1 -> cal1/1(In1)
  Sig1NoTqLoaResp/1 -> cal2/1(In1)
  " "/1 -> HwTqResp/1

== system SF049A_LoaMgr/LoaMgr/LoaMgrPer1/Request_Responses/InvtrResp/CopyRight2 ==

== system SF049A_LoaMgr/LoaMgr/LoaMgrPer1/Request_Responses/InvtrResp/Two ==
  Sig2Resp : Inport
  Two : ActionPort  ActionType=case
  CopyRight2 : Subsystem  Description=|  mask(Copyright Information){none=on}
      | Copyright info block.                                               
      |                                                                     
      | Place copyright information at the top of every subsystem in design.
      mask prompts: none "No parameters"
      mask help: Place copyright information at the top of every subsystem in design.
      mask Display:
      | NxtrConf = 'Nexteer Confidential';
      | 
      | sys = bdroot; %handle for the current model ("system")
      | first = get_param(sys,'Created');
      | first = first(end-3:end);  %year is last four digits
      | 
      | last = get_param(sys,'LastModifiedDate');
      | if isempty(last)
      |     last = datestr(now,'yyyy');
      | else
      |     last = last(end-3:end);
      | end
      | 
      | if strcmp(first,last)
      |     fprintf('%s -- Copyright %s Nexteer',NxtrConf,first)
      | else
      |     fprintf('%s -- %s%s- %s Nexteer',NxtrConf,char(169),first,last)
      | end
  IvtrResp : Outport
  wires:
  Sig2Resp/1 -> IvtrResp/1

== system SF049A_LoaMgr/LoaMgr/LoaMgrPer1/Request_Responses/InvtrResp/Zero_or_Invalid ==
  Sig0Resp : Inport
  Default : ActionPort  ActionType=default
  CopyRight2 : Subsystem  Description=|  mask(Copyright Information){none=on}
      | Copyright info block.                                               
      |                                                                     
      | Place copyright information at the top of every subsystem in design.
      mask prompts: none "No parameters"
      mask help: Place copyright information at the top of every subsystem in design.
      mask Display:
      | NxtrConf = 'Nexteer Confidential';
      | 
      | sys = bdroot; %handle for the current model ("system")
      | first = get_param(sys,'Created');
      | first = first(end-3:end);  %year is last four digits
      | 
      | last = get_param(sys,'LastModifiedDate');
      | if isempty(last)
      |     last = datestr(now,'yyyy');
      | else
      |     last = last(end-3:end);
      | end
      | 
      | if strcmp(first,last)
      |     fprintf('%s -- Copyright %s Nexteer',NxtrConf,first)
      | else
      |     fprintf('%s -- %s%s- %s Nexteer',NxtrConf,char(169),first,last)
      | end
  IvtrResp : Outport
  wires:
  Sig0Resp/1 -> IvtrResp/1

== system SF049A_LoaMgr/LoaMgr/LoaMgrPer1/Request_Responses/InvtrResp/one ==
  Sig1Resp : Inport
  one : ActionPort  ActionType=case
  CopyRight2 : Subsystem  Description=|  mask(Copyright Information){none=on}
      | Copyright info block.                                               
      |                                                                     
      | Place copyright information at the top of every subsystem in design.
      mask prompts: none "No parameters"
      mask help: Place copyright information at the top of every subsystem in design.
      mask Display:
      | NxtrConf = 'Nexteer Confidential';
      | 
      | sys = bdroot; %handle for the current model ("system")
      | first = get_param(sys,'Created');
      | first = first(end-3:end);  %year is last four digits
      | 
      | last = get_param(sys,'LastModifiedDate');
      | if isempty(last)
      |     last = datestr(now,'yyyy');
      | else
      |     last = last(end-3:end);
      | end
      | 
      | if strcmp(first,last)
      |     fprintf('%s -- Copyright %s Nexteer',NxtrConf,first)
      | else
      |     fprintf('%s -- %s%s- %s Nexteer',NxtrConf,char(169),first,last)
      | end
  IvtrResp : Outport
  wires:
  Sig1Resp/1 -> IvtrResp/1

== system SF049A_LoaMgr/LoaMgr/LoaMgrPer1/Request_Responses/MotAgResp/CopyRight2 ==

== system SF049A_LoaMgr/LoaMgr/LoaMgrPer1/Request_Responses/MotAgResp/Three ==
  cal : Inport
  Three : ActionPort  ActionType=case
  CopyRight2 : Subsystem  Description=|  mask(Copyright Information){none=on}
      | Copyright info block.                                               
      |                                                                     
      | Place copyright information at the top of every subsystem in design.
      mask prompts: none "No parameters"
      mask help: Place copyright information at the top of every subsystem in design.
      mask Display:
      | NxtrConf = 'Nexteer Confidential';
      | 
      | sys = bdroot; %handle for the current model ("system")
      | first = get_param(sys,'Created');
      | first = first(end-3:end);  %year is last four digits
      | 
      | last = get_param(sys,'LastModifiedDate');
      | if isempty(last)
      |     last = datestr(now,'yyyy');
      | else
      |     last = last(end-3:end);
      | end
      | 
      | if strcmp(first,last)
      |     fprintf('%s -- Copyright %s Nexteer',NxtrConf,first)
      | else
      |     fprintf('%s -- %s%s- %s Nexteer',NxtrConf,char(169),first,last)
      | end
  MotAgResp : Outport
  wires:
  cal/1 -> MotAgResp/1

== system SF049A_LoaMgr/LoaMgr/LoaMgrPer1/Request_Responses/MotAgResp/Two ==
  cal : Inport
  Two : ActionPort  ActionType=case
  CopyRight2 : Subsystem  Description=|  mask(Copyright Information){none=on}
      | Copyright info block.                                               
      |                                                                     
      | Place copyright information at the top of every subsystem in design.
      mask prompts: none "No parameters"
      mask help: Place copyright information at the top of every subsystem in design.
      mask Display:
      | NxtrConf = 'Nexteer Confidential';
      | 
      | sys = bdroot; %handle for the current model ("system")
      | first = get_param(sys,'Created');
      | first = first(end-3:end);  %year is last four digits
      | 
      | last = get_param(sys,'LastModifiedDate');
      | if isempty(last)
      |     last = datestr(now,'yyyy');
      | else
      |     last = last(end-3:end);
      | end
      | 
      | if strcmp(first,last)
      |     fprintf('%s -- Copyright %s Nexteer',NxtrConf,first)
      | else
      |     fprintf('%s -- %s%s- %s Nexteer',NxtrConf,char(169),first,last)
      | end
  MotAgResp : Outport
  wires:
  cal/1 -> MotAgResp/1

== system SF049A_LoaMgr/LoaMgr/LoaMgrPer1/Request_Responses/MotAgResp/Zero_or_Invalid ==
  MotAgAvlSnsrlsResp : Inport
  MotAgIdptSig0NoResp : Inport  Port=2
  MotAgAvlSnsrls : Inport  Port=3
  Default : ActionPort  ActionType=default
  " " : Merge  RequirementInfo="{'linktype_rmi_doors' '0000bab3 (/E-STEER Core/SubSystem Specifications/Application Functions/SF049A Loss of Assist Manager)' '#SF049A_183' 'true' 'REQ:  SF049A_183' '' } %GIDa_b34ab682_9ee5_4b66_891b_104b2a120ee9"
  CopyRight2 : Subsystem  Description=|  mask(Copyright Information){none=on}
      | Copyright info block.                                               
      |                                                                     
      | Place copyright information at the top of every subsystem in design.
      mask prompts: none "No parameters"
      mask help: Place copyright information at the top of every subsystem in design.
      mask Display:
      | NxtrConf = 'Nexteer Confidential';
      | 
      | sys = bdroot; %handle for the current model ("system")
      | first = get_param(sys,'Created');
      | first = first(end-3:end);  %year is last four digits
      | 
      | last = get_param(sys,'LastModifiedDate');
      | if isempty(last)
      |     last = datestr(now,'yyyy');
      | else
      |     last = last(end-3:end);
      | end
      | 
      | if strcmp(first,last)
      |     fprintf('%s -- Copyright %s Nexteer',NxtrConf,first)
      | else
      |     fprintf('%s -- %s%s- %s Nexteer',NxtrConf,char(169),first,last)
      | end
  Ivtr1Inactv_IF : If  RequirementInfo="{'linktype_rmi_doors' '0000bab3 (/E-STEER Core/SubSystem Specifications/Application Functions/SF049A Loss of Assist Manager)' '#SF049A_183' 'true' 'REQ:  SF049A_183' '' } %GIDa_6bec98c7_1813_4552_97df_1c883a1cde76"  IfExpression=u1
  cal1 : Subsystem  RequirementInfo="{'linktype_rmi_doors' '0000bab3 (/E-STEER Core/SubSystem Specifications/Application Functions/SF049A Loss of Assist Manager)' '#SF049A_183' 'true' 'REQ:  SF049A_183' '' } %GIDa_b4bcc3c8_9ad2_434a_99e5_685748df54cf"  TreatAsAtomicUnit=on
      settings: RTWSystemCode=Inline
  cal2 : Subsystem  RequirementInfo="{'linktype_rmi_doors' '0000bab3 (/E-STEER Core/SubSystem Specifications/Application Functions/SF049A Loss of Assist Manager)' '#SF049A_183' 'true' 'REQ:  SF049A_183' '' } %GIDa_04042943_c496_46a1_a477_1d869c138a23"  TreatAsAtomicUnit=on
      settings: RTWSystemCode=Inline
  MotAgResp : Outport
  wires:
  " "/1 -> MotAgResp/1
  MotAgIdptSig0NoResp/1 -> cal2/1(In1)
  MotAgAvlSnsrlsResp/1 -> cal1/1(In1)
  cal1/1(Out2) -> " "/1
  MotAgAvlSnsrls/1 -> Ivtr1Inactv_IF/1
  cal2/1(Out1) -> " "/2
  Ivtr1Inactv_IF/1 -> cal1/Action
  Ivtr1Inactv_IF/2 -> cal2/Action
